simulink model "Model_1_1"  (R2019b)
settings: Solver=VariableStepAuto  StartTime=0.0  StopTime=10.0  RelTol=1e-3
undefined symbols (not defined in the file or in its folder): alpha_C, alpha_E, alpha_I, beta_C, beta_E, beta_I, c_C, delta, e_0, eta, gamma, mu_t, mu_u, N, P, r, rho
settings Model: Creator=Pål  LastModifiedBy=Pål

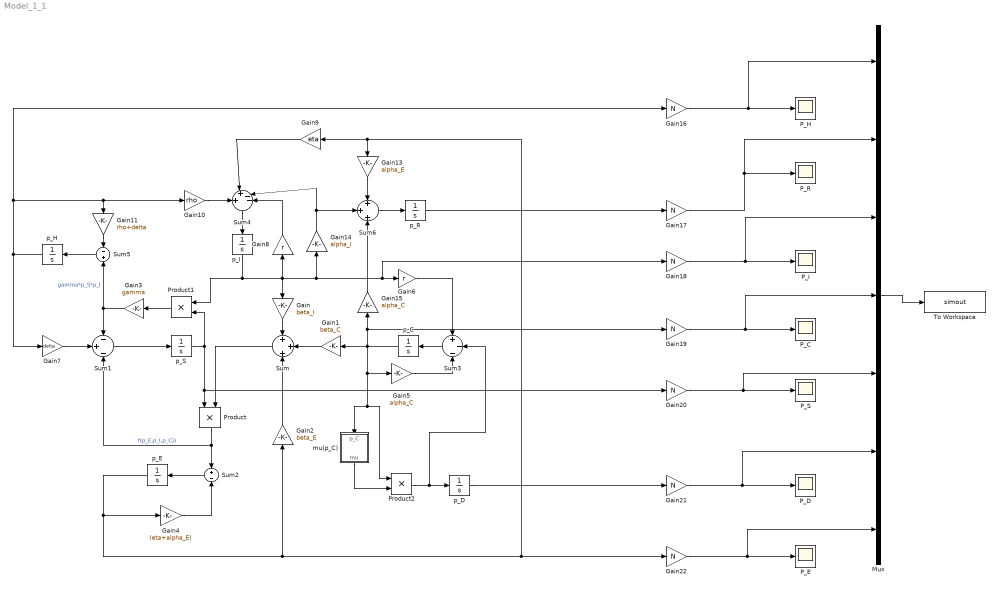
== system Model_1_1 ==
  Gain : Gain  Gain=beta_I
  Gain1 : Gain  Gain=beta_C
  Gain10 : Gain  Gain=rho
  Gain11 : Gain  Gain=rho+delta
  Gain13 : Gain  Gain=alpha_E
  Gain14 : Gain  Gain=alpha_I
  Gain15 : Gain  Gain=alpha_C
  Gain{16..22} (7 alike) : Gain  Gain=N
  Gain2 : Gain  Gain=beta_E
  Gain3 : Gain  Gain=gamma
  Gain4 : Gain  Gain=(eta+alpha_E)
  Gain5 : Gain  Gain=alpha_C
  Gain6 : Gain  Gain=r
  Gain7 : Gain  Gain=delta
  Gain8 : Gain  Gain=r
  Gain9 : Gain  Gain=eta
  Mux : Mux  Inputs=7
  P_C : Scope
  P_D : Scope
  "P_E " : Scope
  P_H : Scope
  P_I : Scope
  "P_R " : Scope
  P_S : Scope
  Product : Product
  Product1 : Product
  Product2 : Product
  Sum : Sum  Inputs=+|+|+
  Sum1 : Sum  Inputs=-|+|-
  Sum2 : Sum  Inputs=+|-
  Sum3 : Sum  Inputs=+|-|-
  Sum4 : Sum  Inputs=+|+|--
  Sum5 : Sum  Inputs=-|+
  Sum6 : Sum  Inputs=+|+|+
  To Workspace : ToWorkspace  VariableName=simout  SaveFormat=Timeseries  SampleTime=-1
  mu(p_C) : Subsystem
  "p_C " : Integrator
  "p_D " : Integrator
  "p_E " : Integrator  InitialCondition=e_0
  p_H : Integrator
  "p_I " : Integrator
  "p_R " : Integrator
  p_S : Integrator  InitialCondition=P
  wires:
  Gain/1 -> Sum/1
  Gain1/1 -> Sum/2
  Gain2/1 -> Sum/3
  Sum/1 -> Product/2
  p_S/1 -> Product1/2, Product/1, Gain20/1
  Product/1 -> Sum2/1, Sum1/3  "f(p_E,p_I,p_C))"
  Sum1/1 -> p_S/1
  Product1/1 -> Gain3/1
  Gain3/1 -> Sum1/1, Sum5/2  "gamma*p_S*p_I"
  "p_I "/1 -> Gain8/1, Gain/1, Gain14/1, Gain18/1, Gain6/1, Product1/1
  Sum2/1 -> "p_E "/1
  "p_E "/1 -> Gain4/1, Gain2/1, Gain22/1, Gain9/1, Gain13/1
  Gain4/1 -> Sum2/2
  "p_C "/1 -> Gain19/1, Gain15/1, Product2/1, mu(p_C)/1(p_C), Gain5/1, Gain1/1
  Sum3/1 -> "p_C "/1
  Gain6/1 -> Sum3/1
  Gain7/1 -> Sum1/2
  p_H/1 -> Gain16/1, Gain11/1, Gain10/1, Gain7/1
  Sum4/1 -> "p_I "/1
  Gain9/1 -> Sum4/2
  Gain10/1 -> Sum4/1
  Sum5/1 -> p_H/1
  Gain11/1 -> Sum5/1
  "p_D "/1 -> Gain21/1
  Sum6/1 -> "p_R "/1
  Gain13/1 -> Sum6/1
  Gain8/1 -> Sum4/4
  Gain14/1 -> Sum6/2, Sum4/3
  Gain15/1 -> Sum6/3
  "p_R "/1 -> Gain17/1
  Gain16/1 -> Mux/1, P_H/1
  Gain22/1 -> Mux/7, "P_E "/1
  Gain21/1 -> Mux/6, P_D/1
  Gain20/1 -> Mux/5, P_S/1
  Gain19/1 -> Mux/4, P_C/1
  Gain18/1 -> P_I/1, Mux/3
  Gain17/1 -> Mux/2, "P_R "/1
  Gain5/1 -> Sum3/3
  Product2/1 -> Sum3/2, "p_D "/1
  mu(p_C)/1(mu) -> Product2/2
  Mux/1 -> To Workspace/1

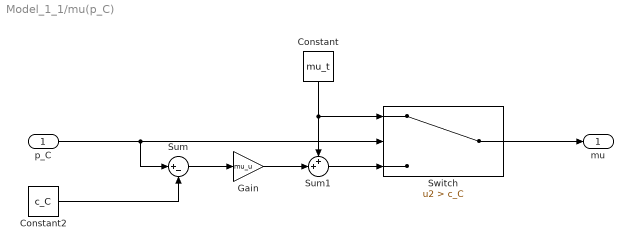
== system Model_1_1/mu(p_C) ==
  p_C : Inport
  Constant : Constant  Value=mu_t
  Constant2 : Constant  Value=c_C
  Gain : Gain  Gain=mu_u
  Sum : Sum  Inputs=|+-
  Sum1 : Sum  Inputs=++|
  Switch : Switch  Criteria=u2 > Threshold  Threshold=c_C
  mu : Outport
  wires:
  p_C/1 -> Sum/1, Switch/2
  Switch/1 -> mu/1
  Constant/1 -> Sum1/1, Switch/1
  Constant2/1 -> Sum/2
  Sum1/1 -> Switch/3
  Gain/1 -> Sum1/2
  Sum/1 -> Gain/1
